simulink model "satellite_11_scenario_2"  (R2021a)
settings: Solver=VariableStepAuto  StartTime=0.0  StopTime=16.0  RelTol=1e-3
undefined symbols (not defined in the file or in its folder): sigbuilder_block
libraries: fuzblock x1
settings Model: Creator=User  LastModifiedBy=User

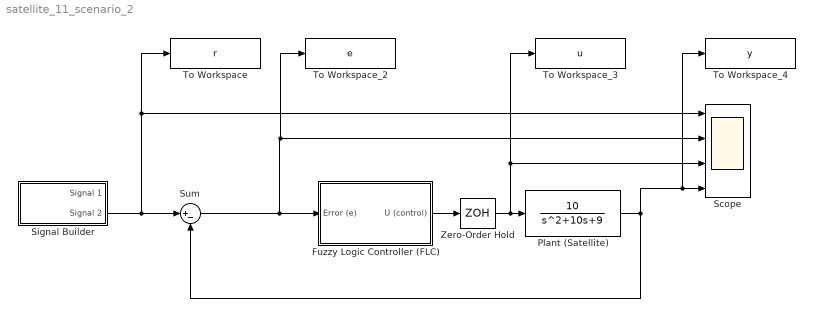
== system satellite_11_scenario_2 ==
  Fuzzy Logic Controller (FLC) : Subsystem
  Plant (Satellite) : TransferFcn  Numerator=[10]  Denominator=[1 10 9]
  "Scope " : Scope  NumInputPorts=4
  Signal Builder : Subsystem  Tag=STV Subsys  LoadFcn=sigbuilder_block('load');  StartFcn=sigbuilder_block('start');  StopFcn=sigbuilder_block('stop');  ClipboardFcn=sigbuilder_block('clipboard');  mask(Sigbuilder block){tuvar=[0:10]}
      mask help: Simulink:masks:SigbuilderBlock_MD
      mask init:
      | if ~strcmp(get_param(bdroot(gcbh),'SimulationStatus'),'stopped') tuvar = sigbuilder_block('maskInit'); end
      settings: CopyFcn=sigbuilder_block('copy');  DeleteFcn=sigbuilder_block('delete');  ModelCloseFcn=sigbuilder_block('modelClose');  PreSaveFcn=sigbuilder_block('preSave');  PauseFcn=sigbuilder_block('pause');  ContinueFcn=sigbuilder_block('continue');  NameChangeFcn=sigbuilder_block('namechange');  OpenFcn=sigbuilder_block('open',[434.4 146.4 550.8 400.2 ]);  CloseFcn=sigbuilder_block('close');
      mask Display: plot(0, 0, 100, 100,[2, 2, 32, 32, 2], [68, 8, 8, 68, 68],[32, 2], [38, 38], [32, 19, 2],[53, 60, 44], [32, 17, 17, 2],[16, 16, 31, 31]);txt = getActiveGroup(gcbh);text(2, 100, txt,'verticalAlignment', 'top');
  Sum : Sum  Inputs=|+-
  "To Workspace " : ToWorkspace  VariableName=r  SaveFormat=Timeseries  SampleTime=-1
  To Workspace_2 : ToWorkspace  VariableName=e  SaveFormat=Timeseries  SampleTime=-1
  To Workspace_3 : ToWorkspace  VariableName=u  SaveFormat=Timeseries  SampleTime=-1
  To Workspace_4 : ToWorkspace  VariableName=y  SaveFormat=Timeseries  SampleTime=-1
  Zero-Order Hold : ZeroOrderHold  SampleTime=-1
  wires:
  Plant (Satellite)/1 -> To Workspace_4/1, "Scope "/4, Sum/2
  Sum/1 -> To Workspace_2/1, "Scope "/2, Fuzzy Logic Controller (FLC)/1(Error (e))
  Fuzzy Logic Controller (FLC)/1("\tU (control)") -> Zero-Order Hold/1
  Zero-Order Hold/1 -> To Workspace_3/1, "Scope "/3, Plant (Satellite)/1
  Signal Builder/2(Signal 2) -> "Scope "/1, "To Workspace "/1, Sum/1

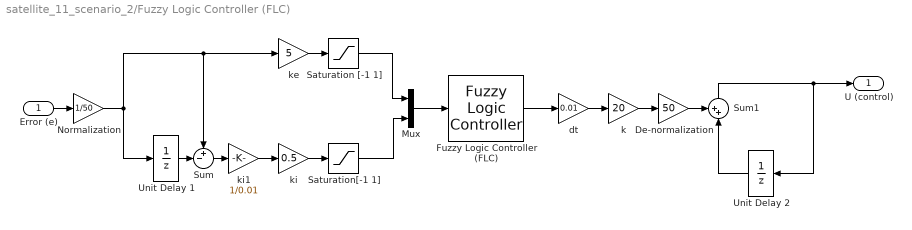
== system satellite_11_scenario_2/Fuzzy Logic Controller (FLC) ==
  Error (e) : Inport
  De-normalization : Gain  Gain=50
  Fuzzy Logic Controller (FLC) : fuzblock/Fuzzy Logic  Controller  FIS='fis_satellite.fis'  OutputSampleNumber=101  DataType=double  FuzzifiedInputs=off  RuleFiringStrengths=off  RuleOutputs=off  AggregatedOutputs=off  SimulateUsing=Interpreted execution  OutOfRangeInputValueMessage=warning  NoRuleFiredMessage=warning  EmptyOutputFuzzySetMessage=warning
  Mux : Mux  Inputs=2
  Normalization : Gain  Gain=1/50
  Saturation [-1 1] : Saturate  UpperLimit=1  LowerLimit=-1
  "Saturation[-1 1] " : Saturate  UpperLimit=1  LowerLimit=-1
  Sum : Sum  Inputs=+-|
  Sum1 : Sum  Inputs=++|
  Unit Delay 1 : UnitDelay  SampleTime=0.01  HasFrameUpgradeWarning=on
  Unit Delay 2 : UnitDelay  SampleTime=0.01  HasFrameUpgradeWarning=on
  dt : Gain  Gain=0.01
  k : Gain  Gain=20
  ke : Gain  Gain=5
  ki : Gain  Gain=0.5
  ki1 : Gain  Gain=1/0.01
  "\tU (control)" : Outport
  wires:
  Error (e)/1 -> Normalization/1
  Fuzzy Logic Controller (FLC)/1 -> dt/1
  Mux/1 -> Fuzzy Logic Controller (FLC)/1
  ki1/1 -> ki/1
  ke/1 -> Saturation [-1 1]/1
  Normalization/1 -> Unit Delay 1/1, Sum/1, ke/1
  Saturation [-1 1]/1 -> Mux/1
  "Saturation[-1 1] "/1 -> Mux/2
  Unit Delay 1/1 -> Sum/2
  Sum/1 -> ki1/1
  De-normalization/1 -> Sum1/1
  Unit Delay 2/1 -> Sum1/2
  ki/1 -> "Saturation[-1 1] "/1
  dt/1 -> k/1
  k/1 -> De-normalization/1
  Sum1/1 -> Unit Delay 2/1, "\tU (control)"/1

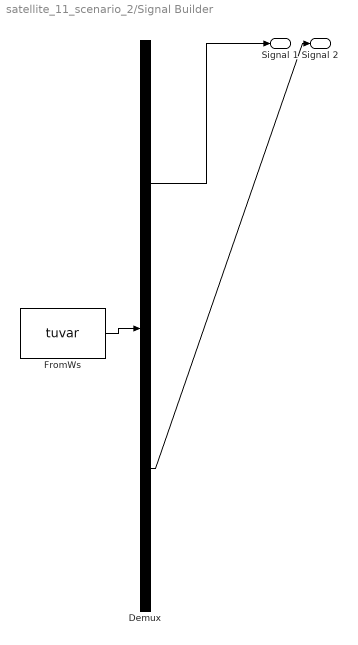
== system satellite_11_scenario_2/Signal Builder ==
  Demux : Demux  Tag=STV Demux  Outputs=2
      settings: DisplayOption=none
  FromWs : FromWorkspace  Tag=STV FromWs  VariableName=tuvar
      SigBuilderData=|
      | common.afterFinalStr = 'Extrapolate'
      | common.sampleTime = 0
      | dataSet.timeRange = [0 16]
      | dataSet.name = 'Group 1'
      | sbobj.Groups.Name = 'Group 1'
      | sbobj.Groups.Signals(1).Name = 'Signal 1'
      | sbobj.Groups.Signals(1).XData = [0 4 4 8 8 16]
      | sbobj.Groups.Signals(1).YData = [60 60 20 20 40 40]
      | sbobj.Groups.Signals(2).Name = 'Signal 2'
      | sbobj.Groups.Signals(2).XData = [0 4 8 16]
      | sbobj.Groups.Signals(2).YData = [0.4 60 60 0.4]
      | sbobj.Groups.TimeRange = [0 16]
  Signal 1 : Outport  Tag=STV Outport
  Signal 2 : Outport  Tag=STV Outport  Port=2
  wires:
  Demux/1 -> Signal 1/1
  FromWs/1 -> Demux/1
  Demux/2 -> Signal 2/1
